simulink model "Crane_rigid"  (R2021b)
settings: Solver=ode15s  StartTime=0.0  StopTime=t_f  MaxStep=max_step_size  RelTol=1e-3
values from neighbouring files (symbols this model uses):
  a_d_full_y = circshift(a_d_full_x,floor(1/h))/2    [modify_tracking.m]
  cont_param_10 = in    [double_pendulum.m]    (also in optimize_10_SMC_single_first_explicit.m = cont_param_10_surrogateopt)
  cont_param_11 = in    [double_pendulum.m]    (also in optimize_11_SMC_single_first_implicit.m = cont_param_11_surrogateopt)
  cont_param_12 = in    [double_pendulum.m]    (also in optimize_12_SMC_single_last_explicit.m = cont_param_12_surrogateopt)
  cont_param_13 = in    [double_pendulum.m]    (also in optimize_13_SMC_single_last_implicit.m = cont_param_13_surrogateopt)
  cont_param_14 = in    [double_pendulum.m]    (also in optimize_14_SMC_double_explicit.m = cont_param_14_surrogateopt)
  cont_param_15 = in    [double_pendulum.m]    (also in optimize_15_SMC_double_implicit.m = cont_param_15_surrogateopt)
  cont_param_16 = in    [double_pendulum.m]
  cont_param_17 = in    [double_pendulum.m]
  cont_param_18 = in    [double_pendulum.m]
  cont_param_19 = in    [double_pendulum.m]
  cont_param_4 = in    [double_pendulum.m]
  cont_param_5 = in    [double_pendulum.m]
  cont_param_6 = in    [double_pendulum.m]
  cont_param_7 = in    [double_pendulum.m]
  cont_param_8 = in    [double_pendulum.m]
  cont_param_9 = in    [double_pendulum.m]
  h = 1e-5    (= 1e-05)    [Conference_paper.m]    (also in Latest.m)
  m = 10    [Conference_paper.m]    (also in Latest.m = 100; control_8_collocated_PD_tracking.m = load_mass+hook_mass+cable_mass_total)
  method_select = Method    [main_run.m]    (also in modify_tracking.m = 3)
  N = floor(t_f / h)    [control_2_zero_vibration.m]    (also in control_3_ZVD.m; modify_tracking.m = 3)
  s = c1*(x-xd)+c2*(v-vd)+c3*theta_dot_1+c4*theta_1    [control_10_SMC_single_first_explicit.m]    (also in control_11_SMC_single_first_implicit.m = c1*(x-xd)+c2*(v-vd)+c3*theta_dot+c4*theta; control_12_SMC_single_last_explicit.m = c1*(x-xd)+c2*(v-vd)+c3*theta_dot_2+c4*theta_2; control_13_SMC_single_last_implicit.m = c1*(x-xd)+c2*(v-vd)+c3*theta_dot+c4*theta; control_14_SMC_double_explicit.m = (v-vd)+lambda*(x-xd)+alpha*theta_1+beta*theta_2)
  sin_traj_w = 0.5    [modify_tracking.m]
  X = ex+lambda*sin(theta)    [control_16_PD_energy_first.m]    (also in control_17_PD_energy_last.m)
  Z = cont_param_8(4)    [control_8_collocated_PD_tracking.m]
undefined symbols (not defined in the file or in its folder): a_d_full_x, all_initial_sway, c_actuator, cable_length, cable_mass_total, cart_disturbance_amp, cart_mass, delay_time, first_link_sway, hook_mass, last_piece_length, load_disturbance_amp, number_of_pendulums, payload_mass, sat_const, sin_traj_A, t_f, total_mass, traj_number, unbalanced_factor, Y
libraries: nesl_utility x180, sm_lib x138, commchan3 x8
(part 2 of 3)

== system Crane_rigid/Rail ==
  F_x : Inport
  F_y : Inport  Port=2
  PS-Simulink Converter{,1..3} (4 alike) : nesl_utility/PS-Simulink Converter  PhysicalDomain=network_engine_domain  SubClassName=ps_output  LeftPortType=input  RightPortType=output  PseudoPeriodic=off  Frequencies=[]  Unit=inherit  AffineConversion=off
      settings: SourceProductBaseCode=PW,SS
  Rectangular Joint : sm_lib/Joints/Rectangular Joint  JointMode=Normal  SenseConstraintForce=off  SenseConstraintForceX=off  SenseConstraintForceY=off  SenseConstraintForceZ=off  SenseConstraintTorque=off  SenseConstraintTorqueX=off  SenseConstraintTorqueY=off  SenseConstraintTorqueZ=off  SenseTotalForce=off  SenseTotalForceX=off  SenseTotalForceY=off  SenseTotalForceZ=off  SenseTotalTorque=off  SenseTotalTorqueX=off  SenseTotalTorqueY=off  SenseTotalTorqueZ=off  CompositeWrenchDir=FollowerOnBase  CompositeWrenchFrame=BaseFrame  PxEquilibriumPosition=0  PxEquilibriumPositionUnits=m  PxSpringStiffness=0  PxSpringStiffnessUnits=N/m  PxDampingCoefficient=0  PxDampingCoefficientUnits=N/(m/s)  PxTorqueActuationMode=InputTorque  PxMotionActuationMode=ComputedMotion  PxSensePosition=off  PxSenseVelocity=off  PxSenseAcceleration=off  PxSenseTorqueForce=off  PxSenseLowerLimitTorqueForce=off  PxSenseUpperLimitTorqueForce=off  PxLowerLimitSpecify=off  PxLowerLimitBound=-1  PxLowerLimitBoundUnits=m  PxLowerLimitStiffness=1e6  PxLowerLimitStiffnessUnits=N/m  PxLowerLimitDamping=1e3  PxLowerLimitDampingUnits=N/(m/s)  PxLowerLimitTransitionRegionWidth=1e-4  PxLowerLimitTransitionRegionWidthUnits=m  PxUpperLimitSpecify=off  PxUpperLimitBound=1  PxUpperLimitBoundUnits=m  PxUpperLimitStiffness=1e6  PxUpperLimitStiffnessUnits=N/m  PxUpperLimitDamping=1e3  PxUpperLimitDampingUnits=N/(m/s)  PxUpperLimitTransitionRegionWidth=1e-4  PxUpperLimitTransitionRegionWidthUnits=m  PxPositionTargetSpecify=off  PxPositionTargetPriority=High  PxPositionTargetValue=0  PxPositionTargetValueUnits=m  PxVelocityTargetSpecify=off  PxVelocityTargetPriority=High  PxVelocityTargetValue=0  PxVelocityTargetValueUnits=m/s  PyEquilibriumPosition=0  PyEquilibriumPositionUnits=m  PySpringStiffness=0  PySpringStiffnessUnits=N/m  PyDampingCoefficient=0  PyDampingCoefficientUnits=N/(m/s)  PyTorqueActuationMode=InputTorque  PyMotionActuationMode=ComputedMotion  PySensePosition=off  PySenseVelocity=off  PySenseAcceleration=off  PySenseTorqueForce=off  PySenseLowerLimitTorqueForce=off  PySenseUpperLimitTorqueForce=off  PyLowerLimitSpecify=off  PyLowerLimitBound=-1  PyLowerLimitBoundUnits=m  PyLowerLimitStiffness=1e6  PyLowerLimitStiffnessUnits=N/m  PyLowerLimitDamping=1e3  PyLowerLimitDampingUnits=N/(m/s)  PyLowerLimitTransitionRegionWidth=1e-4  PyLowerLimitTransitionRegionWidthUnits=m  PyUpperLimitSpecify=off  PyUpperLimitBound=1  PyUpperLimitBoundUnits=m  PyUpperLimitStiffness=1e6  PyUpperLimitStiffnessUnits=N/m  PyUpperLimitDamping=1e3  PyUpperLimitDampingUnits=N/(m/s)  PyUpperLimitTransitionRegionWidth=1e-4  PyUpperLimitTransitionRegionWidthUnits=m  PyPositionTargetSpecify=off  PyPositionTargetPriority=High  PyPositionTargetValue=0  PyPositionTargetValueUnits=m  PyVelocityTargetSpecify=off  PyVelocityTargetPriority=High  PyVelocityTargetValue=0  PyVelocityTargetValueUnits=m/s
  Simulink-PS Converter1 : nesl_utility/Simulink-PS Converter  PhysicalDomain=network_engine_domain  SubClassName=ps_input  LeftPortType=input  RightPortType=output  PseudoPeriodic=off  Frequencies=[]  NoiseDistribution=none  NoiseParameters=[]  Unit=1  AffineConversion=off  FilteringAndDerivatives=provide  SimscapeFilterOrder=1  InputFilterTimeConstant=0.001  UdotUserProvided=0
      settings: SourceProductBaseCode=PW,SS
  Simulink-PS Converter2 : nesl_utility/Simulink-PS Converter  PhysicalDomain=network_engine_domain  SubClassName=ps_input  LeftPortType=input  RightPortType=output  PseudoPeriodic=off  Frequencies=[]  NoiseDistribution=none  NoiseParameters=[]  Unit=1  AffineConversion=off  FilteringAndDerivatives=provide  SimscapeFilterOrder=1  InputFilterTimeConstant=0.001  UdotUserProvided=0
      settings: SourceProductBaseCode=PW,SS
  Transform Sensor : sm_lib/Frames and Transforms/Transform Sensor  MeasurementFrame=World  SenseAngle=off  SenseAxis=off  SenseAngle1=off  SenseAngle2=off  SenseAngle3=off  SenseQ=off  SenseR=off  SenseOmegaX=off  SenseOmegaY=off  SenseOmegaZ=off  SenseOmega1=off  SenseOmega2=off  SenseOmega3=off  SenseQDot=off  SenseRDot=off  SenseAlphaX=off  SenseAlphaY=off  SenseAlphaZ=off  SenseAlpha1=off  SenseAlpha2=off  SenseAlpha3=off  SenseQDDot=off  SenseRDDot=off  SenseX=on  SenseY=on  SenseZ=off  SenseRad=off  SenseAzim=off  SenseDist=off  SenseInc=off  SenseXDot=on  SenseYDot=on  SenseZDot=off  SenseRadDot=off  SenseAzimDot=off  SenseDistDot=off  SenseIncDot=off  SenseXDDot=off  SenseYDDot=off  SenseZDDot=off  SenseRadDDot=off  SenseAzimDDot=off  SenseDistDDot=off  SenseIncDDot=off
  World Frame : sm_lib/Frames and Transforms/World Frame
  Connection Port : PMIOPort  Side=Left
  Connection Port1 : PMIOPort  Port=2  Side=Right
  tag scope: Trolley_position_x=global, Trolley_position_y=global, Trolley_velocity_x=global, Trolley_velocity_y=global
  wires:
  PS-Simulink Converter/1 -> [Trolley_position_x]  "Trolley_position_x"
  PS-Simulink Converter1/1 -> [Trolley_position_y]  "Trolley_position_y"
  PS-Simulink Converter2/1 -> [Trolley_velocity_x]  "Trolley_velocity_x"
  PS-Simulink Converter3/1 -> [Trolley_velocity_y]  "Trolley_velocity_y"
  F_x/1 -> Simulink-PS Converter1/1
  F_y/1 -> Simulink-PS Converter2/1
  connections:
  Connection Port/RConn1 -- Rectangular Joint/LConn1
  Connection Port1/RConn1 -- Rectangular Joint/RConn1 -- Transform Sensor/RConn1
  Transform Sensor/LConn1 -- World Frame/RConn1
  Transform Sensor/RConn2 -- PS-Simulink Converter/LConn1
  Transform Sensor/RConn3 -- PS-Simulink Converter1/LConn1
  Transform Sensor/RConn4 -- PS-Simulink Converter2/LConn1
  Transform Sensor/RConn5 -- PS-Simulink Converter3/LConn1
  Simulink-PS Converter1/RConn1 -- Rectangular Joint/LConn2
  Simulink-PS Converter2/RConn1 -- Rectangular Joint/LConn3

== system Crane_rigid/World Frame ==
  Mechanism Configuration : sm_lib/Utilities/Mechanism Configuration  UniformGravity=Constant  GravityVector=[0 0 -9.80665]  GravityUnits=m/s^2  LinearizationDelta=0.001  JointModeTransitionNonlinearIterations=2
  Solver Configuration : nesl_utility/Solver Configuration  PhysicalDomain=network_engine_domain  SubClassName=solver  LeftPortType=input  RightPortType=generic  Tones=[]  Harmonics=[]  SimulateNoise=off  Profile=off  UseLocalSampling=off  EnableSwitchedLinearOptims=on  FrequencyDomain=off  UseCCode=off  RelTol=0.001  AbsTol=1e-06  MinStep=1e-09  ToWorkspace=off  RevertToSquareIcSolve=off  NumHomotopyIterations=100  PhasorMode=off  PhasorModeNumHarmonics=1  DoDC=off  ResidualTolerance=1e-09  UseLocalSolver=off  LocalSolverChoice=NE_BACKWARD_EULER_ADVANCER  LocalSolverSampleTime=0.001  DoFixedCost=off  MaxNonlinIter=3  MaxModeIter=2  ComputeImpulses=off  ImpulseIterations=2  LinearAlgebra=auto  EquationFormulation=NE_TIME_EF  DelaysMemoryBudget=1024  AutomaticFiltering=on  FilteringTimeConstant=0.001  PartitionStorageMethod=AS_NEEDED  PartitionMemoryBudget=1024  PartitionMethod=ROBUST
      settings: SourceProductBaseCode=PW,SS
  World Frame : sm_lib/Frames and Transforms/World Frame
  Connection Port : PMIOPort  Side=Left
  connections:
  Solver Configuration/RConn1 -- Connection Port/RConn1 -- Mechanism Configuration/RConn1 -- World Frame/RConn1

== system Crane_rigid/trajectory generator ==
  Clock : Clock
  Clock1 : Clock
  Constant : Constant  Value=traj_number
  Constant1 : Constant  Value=traj_number
  Constant2 : Constant  Value=sin_traj_w
  Constant3 : Constant  Value=sin_traj_A
  Constant4 : Constant  Value=sin_traj_w
  Constant5 : Constant  Value=sin_traj_A
  Gain : Gain  Gain=0.5
  Gain1 : Gain  Gain=0.5
  Gain2 : Gain  Gain=0.5
  Transport Delay : TransportDelay
  Transport Delay1 : TransportDelay
  Transport Delay2 : TransportDelay
  traj1_y : MATLAB Function  TreatAsAtomicUnit=on
  traj_x : MATLAB Function  TreatAsAtomicUnit=on
  tag scope: xd=global, xd_ddot=global, xd_dot=global, yd=global, yd_ddot=global, yd_dot=global
  wires:
  traj_x/1(x_d) -> [xd]  "xd"
  Clock/1 -> traj_x/1(t)
  traj_x/2(v_d) -> [xd_dot]  "xd_dot"
  traj_x/3(a_d) -> [xd_ddot]  "xd_ddot"
  Constant/1 -> traj_x/2(traj_number)
  traj1_y/3(a_d) -> Gain2/1
  traj1_y/2(v_d) -> Gain1/1
  traj1_y/1(x_d) -> Gain/1
  Gain/1 -> Transport Delay/1
  Transport Delay/1 -> [yd]  "yd"
  Gain1/1 -> Transport Delay1/1
  Transport Delay1/1 -> [yd_dot]  "yd_dot"
  Gain2/1 -> Transport Delay2/1
  Transport Delay2/1 -> [yd_ddot]  "yd_ddot"
  Constant2/1 -> traj_x/3(sin_traj_w)
  Constant3/1 -> traj_x/4(sin_traj_A)
  Constant5/1 -> traj1_y/4(sin_traj_A)
  Constant4/1 -> traj1_y/3(sin_traj_w)
  Constant1/1 -> traj1_y/2(traj_number)
  Clock1/1 -> traj1_y/1(t)

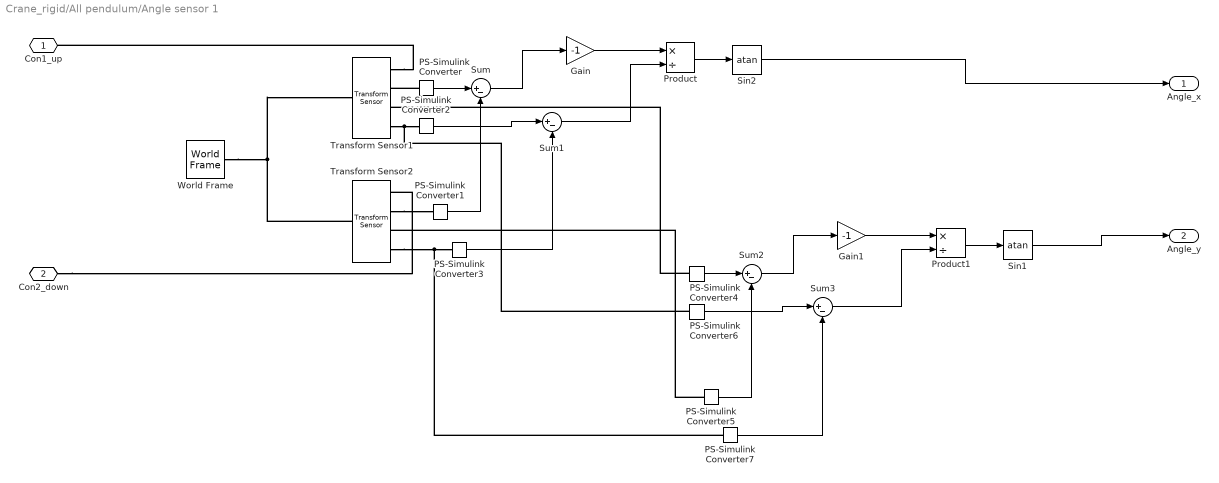
== system Crane_rigid/All pendulum/Angle sensor 1 ==
  Gain : Gain  Gain=-1
  Gain1 : Gain  Gain=-1
  PS-Simulink Converter{,1..7} (8 alike) : nesl_utility/PS-Simulink Converter  PhysicalDomain=network_engine_domain  SubClassName=ps_output  LeftPortType=input  RightPortType=output  PseudoPeriodic=off  Frequencies=[]  Unit=inherit  AffineConversion=off
      settings: SourceProductBaseCode=PW,SS
  Product : Product  Inputs=*/
  Product1 : Product  Inputs=*/
  Sin1 : Trigonometry  Operator=atan
  Sin2 : Trigonometry  Operator=atan
  Sum{,1..3} (4 alike) : Sum  Inputs=|+-
  Transform Sensor1 : sm_lib/Frames and Transforms/Transform Sensor  MeasurementFrame=World  SenseAngle=off  SenseAxis=off  SenseAngle1=off  SenseAngle2=off  SenseAngle3=off  SenseQ=off  SenseR=off  SenseOmegaX=off  SenseOmegaY=off  SenseOmegaZ=off  SenseOmega1=off  SenseOmega2=off  SenseOmega3=off  SenseQDot=off  SenseRDot=off  SenseAlphaX=off  SenseAlphaY=off  SenseAlphaZ=off  SenseAlpha1=off  SenseAlpha2=off  SenseAlpha3=off  SenseQDDot=off  SenseRDDot=off  SenseX=on  SenseY=on  SenseZ=on  SenseRad=off  SenseAzim=off  SenseDist=off  SenseInc=off  SenseXDot=off  SenseYDot=off  SenseZDot=off  SenseRadDot=off  SenseAzimDot=off  SenseDistDot=off  SenseIncDot=off  SenseXDDot=off  SenseYDDot=off  SenseZDDot=off  SenseRadDDot=off  SenseAzimDDot=off  SenseDistDDot=off  SenseIncDDot=off
  Transform Sensor2 : sm_lib/Frames and Transforms/Transform Sensor  MeasurementFrame=World  SenseAngle=off  SenseAxis=off  SenseAngle1=off  SenseAngle2=off  SenseAngle3=off  SenseQ=off  SenseR=off  SenseOmegaX=off  SenseOmegaY=off  SenseOmegaZ=off  SenseOmega1=off  SenseOmega2=off  SenseOmega3=off  SenseQDot=off  SenseRDot=off  SenseAlphaX=off  SenseAlphaY=off  SenseAlphaZ=off  SenseAlpha1=off  SenseAlpha2=off  SenseAlpha3=off  SenseQDDot=off  SenseRDDot=off  SenseX=on  SenseY=on  SenseZ=on  SenseRad=off  SenseAzim=off  SenseDist=off  SenseInc=off  SenseXDot=off  SenseYDot=off  SenseZDot=off  SenseRadDot=off  SenseAzimDot=off  SenseDistDot=off  SenseIncDot=off  SenseXDDot=off  SenseYDDot=off  SenseZDDot=off  SenseRadDDot=off  SenseAzimDDot=off  SenseDistDDot=off  SenseIncDDot=off
  World Frame : sm_lib/Frames and Transforms/World Frame
  Con1_up : PMIOPort  Side=Left
  Con2_down : PMIOPort  Port=2  Side=Left
  Angle_x : Outport
  Angle_y : Outport  Port=2
  wires:
  PS-Simulink Converter/1 -> Sum/1
  Sum1/1 -> Product/2
  Product/1 -> Sin2/1
  PS-Simulink Converter2/1 -> Sum1/1
  PS-Simulink Converter3/1 -> Sum1/2
  Gain/1 -> Product/1
  PS-Simulink Converter7/1 -> Sum3/2
  PS-Simulink Converter4/1 -> Sum2/1
  PS-Simulink Converter5/1 -> Sum2/2
  PS-Simulink Converter1/1 -> Sum/2
  PS-Simulink Converter6/1 -> Sum3/1
  Product1/1 -> Sin1/1
  Sum2/1 -> Gain1/1
  Sum3/1 -> Product1/2
  Gain1/1 -> Product1/1
  Sum/1 -> Gain/1
  Sin2/1 -> Angle_x/1
  Sin1/1 -> Angle_y/1
  connections:
  World Frame/RConn1 -- Transform Sensor2/LConn1 -- Transform Sensor1/LConn1
  Transform Sensor2/RConn4 -- PS-Simulink Converter7/LConn1 -- PS-Simulink Converter3/LConn1
  Transform Sensor1/RConn4 -- PS-Simulink Converter6/LConn1 -- PS-Simulink Converter2/LConn1
  PS-Simulink Converter5/LConn1 -- Transform Sensor2/RConn3
  PS-Simulink Converter4/LConn1 -- Transform Sensor1/RConn3
  Transform Sensor2/RConn2 -- PS-Simulink Converter1/LConn1
  PS-Simulink Converter/LConn1 -- Transform Sensor1/RConn2
  Transform Sensor1/RConn1 -- Con1_up/RConn1
  Con2_down/RConn1 -- Transform Sensor2/RConn1

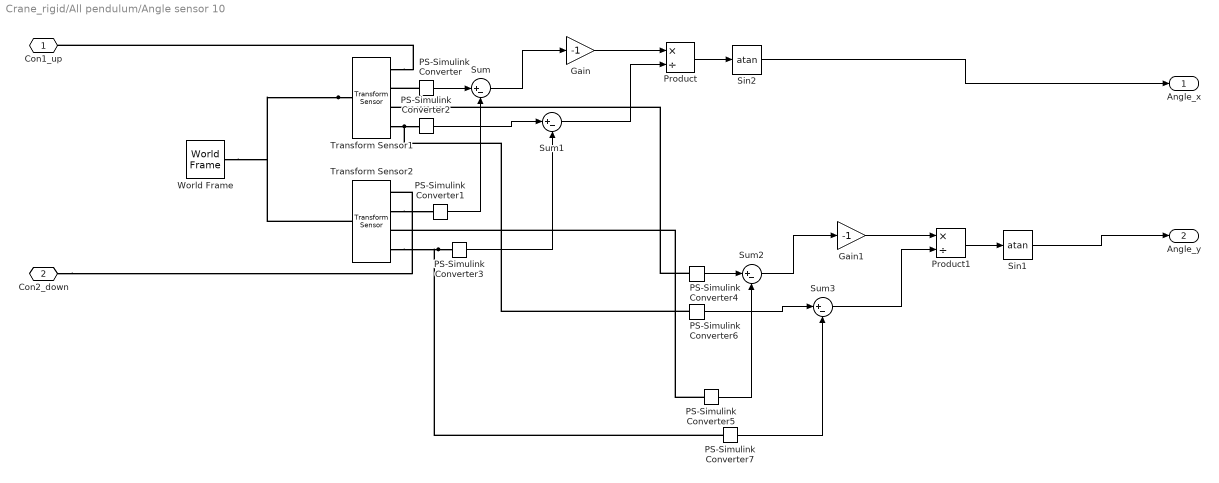
== system Crane_rigid/All pendulum/Angle sensor 10 ==
  Gain : Gain  Gain=-1
  Gain1 : Gain  Gain=-1
  PS-Simulink Converter{,1..7} (8 alike) : nesl_utility/PS-Simulink Converter  PhysicalDomain=network_engine_domain  SubClassName=ps_output  LeftPortType=input  RightPortType=output  PseudoPeriodic=off  Frequencies=[]  Unit=inherit  AffineConversion=off
      settings: SourceProductBaseCode=PW,SS
  Product : Product  Inputs=*/
  Product1 : Product  Inputs=*/
  Sin1 : Trigonometry  Operator=atan
  Sin2 : Trigonometry  Operator=atan
  Sum{,1..3} (4 alike) : Sum  Inputs=|+-
  Transform Sensor1 : sm_lib/Frames and Transforms/Transform Sensor  MeasurementFrame=World  SenseAngle=off  SenseAxis=off  SenseAngle1=off  SenseAngle2=off  SenseAngle3=off  SenseQ=off  SenseR=off  SenseOmegaX=off  SenseOmegaY=off  SenseOmegaZ=off  SenseOmega1=off  SenseOmega2=off  SenseOmega3=off  SenseQDot=off  SenseRDot=off  SenseAlphaX=off  SenseAlphaY=off  SenseAlphaZ=off  SenseAlpha1=off  SenseAlpha2=off  SenseAlpha3=off  SenseQDDot=off  SenseRDDot=off  SenseX=on  SenseY=on  SenseZ=on  SenseRad=off  SenseAzim=off  SenseDist=off  SenseInc=off  SenseXDot=off  SenseYDot=off  SenseZDot=off  SenseRadDot=off  SenseAzimDot=off  SenseDistDot=off  SenseIncDot=off  SenseXDDot=off  SenseYDDot=off  SenseZDDot=off  SenseRadDDot=off  SenseAzimDDot=off  SenseDistDDot=off  SenseIncDDot=off
  Transform Sensor2 : sm_lib/Frames and Transforms/Transform Sensor  MeasurementFrame=World  SenseAngle=off  SenseAxis=off  SenseAngle1=off  SenseAngle2=off  SenseAngle3=off  SenseQ=off  SenseR=off  SenseOmegaX=off  SenseOmegaY=off  SenseOmegaZ=off  SenseOmega1=off  SenseOmega2=off  SenseOmega3=off  SenseQDot=off  SenseRDot=off  SenseAlphaX=off  SenseAlphaY=off  SenseAlphaZ=off  SenseAlpha1=off  SenseAlpha2=off  SenseAlpha3=off  SenseQDDot=off  SenseRDDot=off  SenseX=on  SenseY=on  SenseZ=on  SenseRad=off  SenseAzim=off  SenseDist=off  SenseInc=off  SenseXDot=off  SenseYDot=off  SenseZDot=off  SenseRadDot=off  SenseAzimDot=off  SenseDistDot=off  SenseIncDot=off  SenseXDDot=off  SenseYDDot=off  SenseZDDot=off  SenseRadDDot=off  SenseAzimDDot=off  SenseDistDDot=off  SenseIncDDot=off
  World Frame : sm_lib/Frames and Transforms/World Frame
  Con1_up : PMIOPort  Side=Left
  Con2_down : PMIOPort  Port=2  Side=Left
  Angle_x : Outport
  Angle_y : Outport  Port=2
  wires:
  Sin1/1 -> Angle_y/1
  Sin2/1 -> Angle_x/1
  Sum/1 -> Gain/1
  Gain1/1 -> Product1/1
  Sum3/1 -> Product1/2
  Sum2/1 -> Gain1/1
  Product1/1 -> Sin1/1
  PS-Simulink Converter6/1 -> Sum3/1
  PS-Simulink Converter1/1 -> Sum/2
  PS-Simulink Converter5/1 -> Sum2/2
  PS-Simulink Converter4/1 -> Sum2/1
  PS-Simulink Converter7/1 -> Sum3/2
  Gain/1 -> Product/1
  PS-Simulink Converter3/1 -> Sum1/2
  PS-Simulink Converter2/1 -> Sum1/1
  Product/1 -> Sin2/1
  Sum1/1 -> Product/2
  PS-Simulink Converter/1 -> Sum/1
  connections:
  Con2_down/RConn1 -- Transform Sensor2/RConn1
  Transform Sensor1/RConn1 -- Con1_up/RConn1
  PS-Simulink Converter/LConn1 -- Transform Sensor1/RConn2
  Transform Sensor2/RConn2 -- PS-Simulink Converter1/LConn1
  PS-Simulink Converter4/LConn1 -- Transform Sensor1/RConn3
  PS-Simulink Converter5/LConn1 -- Transform Sensor2/RConn3
  PS-Simulink Converter2/LConn1 -- PS-Simulink Converter6/LConn1 -- Transform Sensor1/RConn4
  PS-Simulink Converter3/LConn1 -- PS-Simulink Converter7/LConn1 -- Transform Sensor2/RConn4
  Transform Sensor1/LConn1 -- Transform Sensor2/LConn1 -- World Frame/RConn1

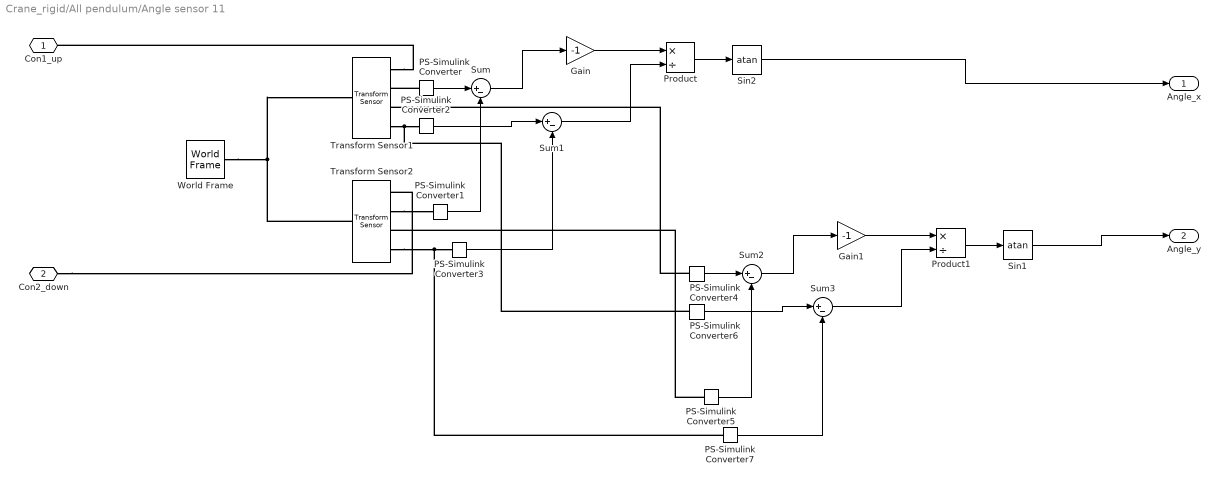
== system Crane_rigid/All pendulum/Angle sensor 11 ==
  Gain : Gain  Gain=-1
  Gain1 : Gain  Gain=-1
  PS-Simulink Converter{,1..7} (8 alike) : nesl_utility/PS-Simulink Converter  PhysicalDomain=network_engine_domain  SubClassName=ps_output  LeftPortType=input  RightPortType=output  PseudoPeriodic=off  Frequencies=[]  Unit=inherit  AffineConversion=off
      settings: SourceProductBaseCode=PW,SS
  Product : Product  Inputs=*/
  Product1 : Product  Inputs=*/
  Sin1 : Trigonometry  Operator=atan
  Sin2 : Trigonometry  Operator=atan
  Sum{,1..3} (4 alike) : Sum  Inputs=|+-
  Transform Sensor1 : sm_lib/Frames and Transforms/Transform Sensor  MeasurementFrame=World  SenseAngle=off  SenseAxis=off  SenseAngle1=off  SenseAngle2=off  SenseAngle3=off  SenseQ=off  SenseR=off  SenseOmegaX=off  SenseOmegaY=off  SenseOmegaZ=off  SenseOmega1=off  SenseOmega2=off  SenseOmega3=off  SenseQDot=off  SenseRDot=off  SenseAlphaX=off  SenseAlphaY=off  SenseAlphaZ=off  SenseAlpha1=off  SenseAlpha2=off  SenseAlpha3=off  SenseQDDot=off  SenseRDDot=off  SenseX=on  SenseY=on  SenseZ=on  SenseRad=off  SenseAzim=off  SenseDist=off  SenseInc=off  SenseXDot=off  SenseYDot=off  SenseZDot=off  SenseRadDot=off  SenseAzimDot=off  SenseDistDot=off  SenseIncDot=off  SenseXDDot=off  SenseYDDot=off  SenseZDDot=off  SenseRadDDot=off  SenseAzimDDot=off  SenseDistDDot=off  SenseIncDDot=off
  Transform Sensor2 : sm_lib/Frames and Transforms/Transform Sensor  MeasurementFrame=World  SenseAngle=off  SenseAxis=off  SenseAngle1=off  SenseAngle2=off  SenseAngle3=off  SenseQ=off  SenseR=off  SenseOmegaX=off  SenseOmegaY=off  SenseOmegaZ=off  SenseOmega1=off  SenseOmega2=off  SenseOmega3=off  SenseQDot=off  SenseRDot=off  SenseAlphaX=off  SenseAlphaY=off  SenseAlphaZ=off  SenseAlpha1=off  SenseAlpha2=off  SenseAlpha3=off  SenseQDDot=off  SenseRDDot=off  SenseX=on  SenseY=on  SenseZ=on  SenseRad=off  SenseAzim=off  SenseDist=off  SenseInc=off  SenseXDot=off  SenseYDot=off  SenseZDot=off  SenseRadDot=off  SenseAzimDot=off  SenseDistDot=off  SenseIncDot=off  SenseXDDot=off  SenseYDDot=off  SenseZDDot=off  SenseRadDDot=off  SenseAzimDDot=off  SenseDistDDot=off  SenseIncDDot=off
  World Frame : sm_lib/Frames and Transforms/World Frame
  Con1_up : PMIOPort  Side=Left
  Con2_down : PMIOPort  Port=2  Side=Left
  Angle_x : Outport
  Angle_y : Outport  Port=2
  wires:
  PS-Simulink Converter/1 -> Sum/1
  Sum1/1 -> Product/2
  Product/1 -> Sin2/1
  PS-Simulink Converter2/1 -> Sum1/1
  PS-Simulink Converter3/1 -> Sum1/2
  Gain/1 -> Product/1
  PS-Simulink Converter7/1 -> Sum3/2
  PS-Simulink Converter4/1 -> Sum2/1
  PS-Simulink Converter5/1 -> Sum2/2
  PS-Simulink Converter1/1 -> Sum/2
  PS-Simulink Converter6/1 -> Sum3/1
  Product1/1 -> Sin1/1
  Sum2/1 -> Gain1/1
  Sum3/1 -> Product1/2
  Gain1/1 -> Product1/1
  Sum/1 -> Gain/1
  Sin2/1 -> Angle_x/1
  Sin1/1 -> Angle_y/1
  connections:
  World Frame/RConn1 -- Transform Sensor2/LConn1 -- Transform Sensor1/LConn1
  Transform Sensor2/RConn4 -- PS-Simulink Converter7/LConn1 -- PS-Simulink Converter3/LConn1
  Transform Sensor1/RConn4 -- PS-Simulink Converter6/LConn1 -- PS-Simulink Converter2/LConn1
  PS-Simulink Converter5/LConn1 -- Transform Sensor2/RConn3
  PS-Simulink Converter4/LConn1 -- Transform Sensor1/RConn3
  Transform Sensor2/RConn2 -- PS-Simulink Converter1/LConn1
  PS-Simulink Converter/LConn1 -- Transform Sensor1/RConn2
  Transform Sensor1/RConn1 -- Con1_up/RConn1
  Con2_down/RConn1 -- Transform Sensor2/RConn1

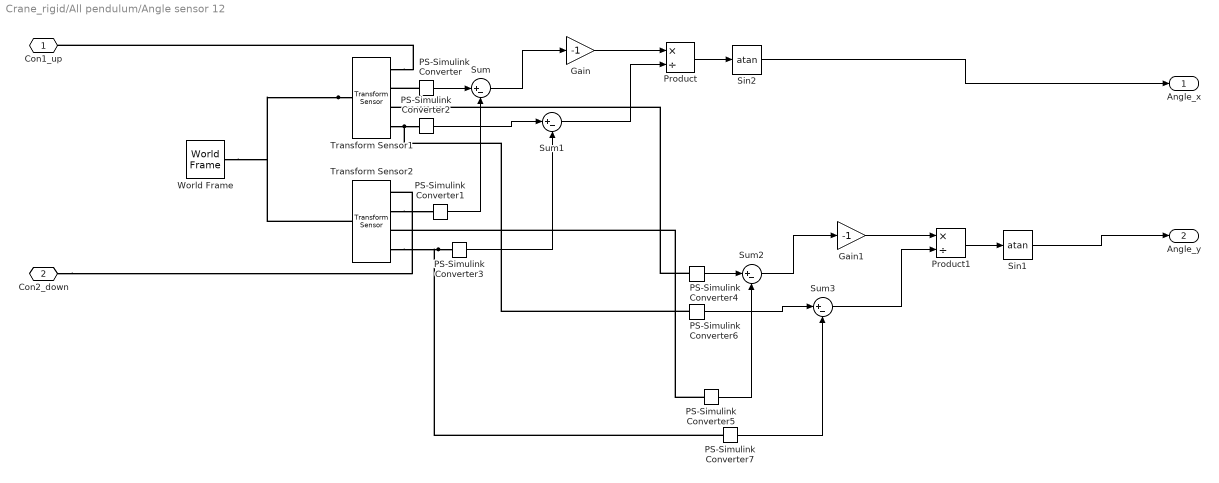
== system Crane_rigid/All pendulum/Angle sensor 12 ==
  Gain : Gain  Gain=-1
  Gain1 : Gain  Gain=-1
  PS-Simulink Converter{,1..7} (8 alike) : nesl_utility/PS-Simulink Converter  PhysicalDomain=network_engine_domain  SubClassName=ps_output  LeftPortType=input  RightPortType=output  PseudoPeriodic=off  Frequencies=[]  Unit=inherit  AffineConversion=off
      settings: SourceProductBaseCode=PW,SS
  Product : Product  Inputs=*/
  Product1 : Product  Inputs=*/
  Sin1 : Trigonometry  Operator=atan
  Sin2 : Trigonometry  Operator=atan
  Sum{,1..3} (4 alike) : Sum  Inputs=|+-
  Transform Sensor1 : sm_lib/Frames and Transforms/Transform Sensor  MeasurementFrame=World  SenseAngle=off  SenseAxis=off  SenseAngle1=off  SenseAngle2=off  SenseAngle3=off  SenseQ=off  SenseR=off  SenseOmegaX=off  SenseOmegaY=off  SenseOmegaZ=off  SenseOmega1=off  SenseOmega2=off  SenseOmega3=off  SenseQDot=off  SenseRDot=off  SenseAlphaX=off  SenseAlphaY=off  SenseAlphaZ=off  SenseAlpha1=off  SenseAlpha2=off  SenseAlpha3=off  SenseQDDot=off  SenseRDDot=off  SenseX=on  SenseY=on  SenseZ=on  SenseRad=off  SenseAzim=off  SenseDist=off  SenseInc=off  SenseXDot=off  SenseYDot=off  SenseZDot=off  SenseRadDot=off  SenseAzimDot=off  SenseDistDot=off  SenseIncDot=off  SenseXDDot=off  SenseYDDot=off  SenseZDDot=off  SenseRadDDot=off  SenseAzimDDot=off  SenseDistDDot=off  SenseIncDDot=off
  Transform Sensor2 : sm_lib/Frames and Transforms/Transform Sensor  MeasurementFrame=World  SenseAngle=off  SenseAxis=off  SenseAngle1=off  SenseAngle2=off  SenseAngle3=off  SenseQ=off  SenseR=off  SenseOmegaX=off  SenseOmegaY=off  SenseOmegaZ=off  SenseOmega1=off  SenseOmega2=off  SenseOmega3=off  SenseQDot=off  SenseRDot=off  SenseAlphaX=off  SenseAlphaY=off  SenseAlphaZ=off  SenseAlpha1=off  SenseAlpha2=off  SenseAlpha3=off  SenseQDDot=off  SenseRDDot=off  SenseX=on  SenseY=on  SenseZ=on  SenseRad=off  SenseAzim=off  SenseDist=off  SenseInc=off  SenseXDot=off  SenseYDot=off  SenseZDot=off  SenseRadDot=off  SenseAzimDot=off  SenseDistDot=off  SenseIncDot=off  SenseXDDot=off  SenseYDDot=off  SenseZDDot=off  SenseRadDDot=off  SenseAzimDDot=off  SenseDistDDot=off  SenseIncDDot=off
  World Frame : sm_lib/Frames and Transforms/World Frame
  Con1_up : PMIOPort  Side=Left
  Con2_down : PMIOPort  Port=2  Side=Left
  Angle_x : Outport
  Angle_y : Outport  Port=2
  wires:
  Sin1/1 -> Angle_y/1
  Sin2/1 -> Angle_x/1
  Sum/1 -> Gain/1
  Gain1/1 -> Product1/1
  Sum3/1 -> Product1/2
  Sum2/1 -> Gain1/1
  Product1/1 -> Sin1/1
  PS-Simulink Converter6/1 -> Sum3/1
  PS-Simulink Converter1/1 -> Sum/2
  PS-Simulink Converter5/1 -> Sum2/2
  PS-Simulink Converter4/1 -> Sum2/1
  PS-Simulink Converter7/1 -> Sum3/2
  Gain/1 -> Product/1
  PS-Simulink Converter3/1 -> Sum1/2
  PS-Simulink Converter2/1 -> Sum1/1
  Product/1 -> Sin2/1
  Sum1/1 -> Product/2
  PS-Simulink Converter/1 -> Sum/1
  connections:
  Con2_down/RConn1 -- Transform Sensor2/RConn1
  Transform Sensor1/RConn1 -- Con1_up/RConn1
  PS-Simulink Converter/LConn1 -- Transform Sensor1/RConn2
  Transform Sensor2/RConn2 -- PS-Simulink Converter1/LConn1
  PS-Simulink Converter4/LConn1 -- Transform Sensor1/RConn3
  PS-Simulink Converter5/LConn1 -- Transform Sensor2/RConn3
  PS-Simulink Converter2/LConn1 -- PS-Simulink Converter6/LConn1 -- Transform Sensor1/RConn4
  PS-Simulink Converter3/LConn1 -- PS-Simulink Converter7/LConn1 -- Transform Sensor2/RConn4
  Transform Sensor1/LConn1 -- Transform Sensor2/LConn1 -- World Frame/RConn1

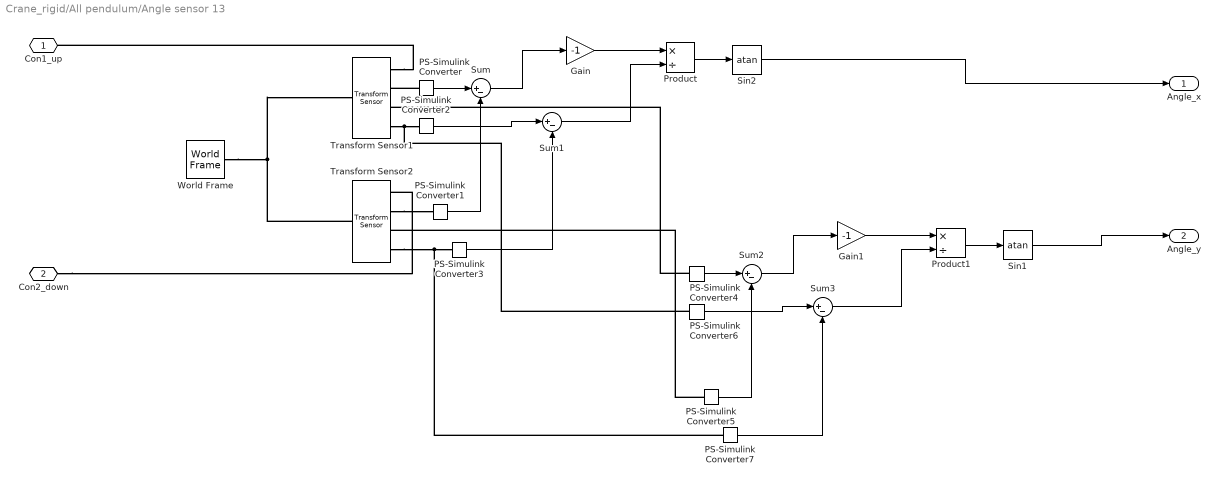
== system Crane_rigid/All pendulum/Angle sensor 13 ==
  Gain : Gain  Gain=-1
  Gain1 : Gain  Gain=-1
  PS-Simulink Converter{,1..7} (8 alike) : nesl_utility/PS-Simulink Converter  PhysicalDomain=network_engine_domain  SubClassName=ps_output  LeftPortType=input  RightPortType=output  PseudoPeriodic=off  Frequencies=[]  Unit=inherit  AffineConversion=off
      settings: SourceProductBaseCode=PW,SS
  Product : Product  Inputs=*/
  Product1 : Product  Inputs=*/
  Sin1 : Trigonometry  Operator=atan
  Sin2 : Trigonometry  Operator=atan
  Sum{,1..3} (4 alike) : Sum  Inputs=|+-
  Transform Sensor1 : sm_lib/Frames and Transforms/Transform Sensor  MeasurementFrame=World  SenseAngle=off  SenseAxis=off  SenseAngle1=off  SenseAngle2=off  SenseAngle3=off  SenseQ=off  SenseR=off  SenseOmegaX=off  SenseOmegaY=off  SenseOmegaZ=off  SenseOmega1=off  SenseOmega2=off  SenseOmega3=off  SenseQDot=off  SenseRDot=off  SenseAlphaX=off  SenseAlphaY=off  SenseAlphaZ=off  SenseAlpha1=off  SenseAlpha2=off  SenseAlpha3=off  SenseQDDot=off  SenseRDDot=off  SenseX=on  SenseY=on  SenseZ=on  SenseRad=off  SenseAzim=off  SenseDist=off  SenseInc=off  SenseXDot=off  SenseYDot=off  SenseZDot=off  SenseRadDot=off  SenseAzimDot=off  SenseDistDot=off  SenseIncDot=off  SenseXDDot=off  SenseYDDot=off  SenseZDDot=off  SenseRadDDot=off  SenseAzimDDot=off  SenseDistDDot=off  SenseIncDDot=off
  Transform Sensor2 : sm_lib/Frames and Transforms/Transform Sensor  MeasurementFrame=World  SenseAngle=off  SenseAxis=off  SenseAngle1=off  SenseAngle2=off  SenseAngle3=off  SenseQ=off  SenseR=off  SenseOmegaX=off  SenseOmegaY=off  SenseOmegaZ=off  SenseOmega1=off  SenseOmega2=off  SenseOmega3=off  SenseQDot=off  SenseRDot=off  SenseAlphaX=off  SenseAlphaY=off  SenseAlphaZ=off  SenseAlpha1=off  SenseAlpha2=off  SenseAlpha3=off  SenseQDDot=off  SenseRDDot=off  SenseX=on  SenseY=on  SenseZ=on  SenseRad=off  SenseAzim=off  SenseDist=off  SenseInc=off  SenseXDot=off  SenseYDot=off  SenseZDot=off  SenseRadDot=off  SenseAzimDot=off  SenseDistDot=off  SenseIncDot=off  SenseXDDot=off  SenseYDDot=off  SenseZDDot=off  SenseRadDDot=off  SenseAzimDDot=off  SenseDistDDot=off  SenseIncDDot=off
  World Frame : sm_lib/Frames and Transforms/World Frame
  Con1_up : PMIOPort  Side=Left
  Con2_down : PMIOPort  Port=2  Side=Left
  Angle_x : Outport
  Angle_y : Outport  Port=2
  wires:
  PS-Simulink Converter/1 -> Sum/1
  Sum1/1 -> Product/2
  Product/1 -> Sin2/1
  PS-Simulink Converter2/1 -> Sum1/1
  PS-Simulink Converter3/1 -> Sum1/2
  Gain/1 -> Product/1
  PS-Simulink Converter7/1 -> Sum3/2
  PS-Simulink Converter4/1 -> Sum2/1
  PS-Simulink Converter5/1 -> Sum2/2
  PS-Simulink Converter1/1 -> Sum/2
  PS-Simulink Converter6/1 -> Sum3/1
  Product1/1 -> Sin1/1
  Sum2/1 -> Gain1/1
  Sum3/1 -> Product1/2
  Gain1/1 -> Product1/1
  Sum/1 -> Gain/1
  Sin2/1 -> Angle_x/1
  Sin1/1 -> Angle_y/1
  connections:
  World Frame/RConn1 -- Transform Sensor2/LConn1 -- Transform Sensor1/LConn1
  Transform Sensor2/RConn4 -- PS-Simulink Converter7/LConn1 -- PS-Simulink Converter3/LConn1
  Transform Sensor1/RConn4 -- PS-Simulink Converter6/LConn1 -- PS-Simulink Converter2/LConn1
  PS-Simulink Converter5/LConn1 -- Transform Sensor2/RConn3
  PS-Simulink Converter4/LConn1 -- Transform Sensor1/RConn3
  Transform Sensor2/RConn2 -- PS-Simulink Converter1/LConn1
  PS-Simulink Converter/LConn1 -- Transform Sensor1/RConn2
  Transform Sensor1/RConn1 -- Con1_up/RConn1
  Con2_down/RConn1 -- Transform Sensor2/RConn1

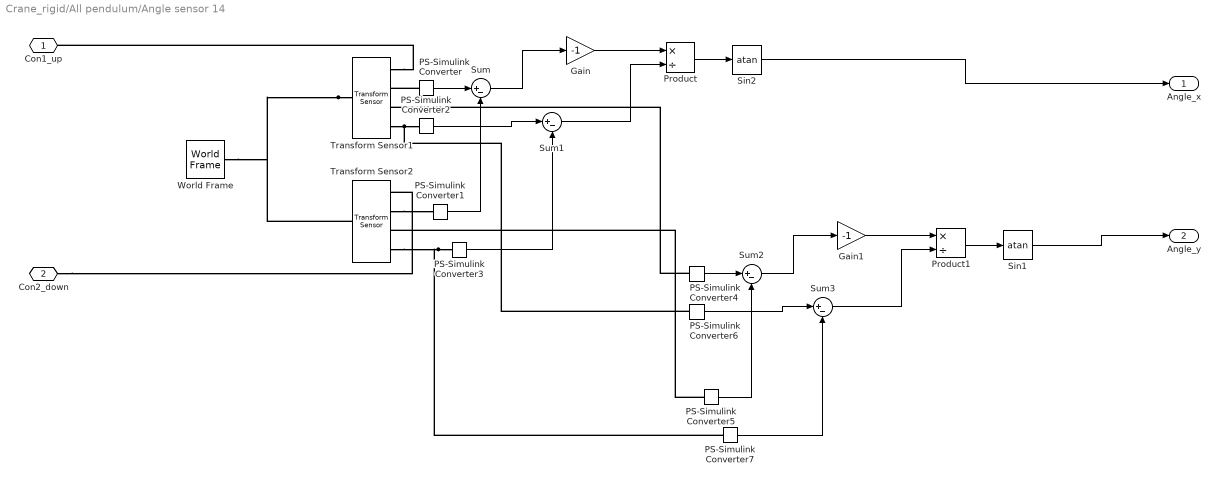
== system Crane_rigid/All pendulum/Angle sensor 14 ==
  Gain : Gain  Gain=-1
  Gain1 : Gain  Gain=-1
  PS-Simulink Converter{,1..7} (8 alike) : nesl_utility/PS-Simulink Converter  PhysicalDomain=network_engine_domain  SubClassName=ps_output  LeftPortType=input  RightPortType=output  PseudoPeriodic=off  Frequencies=[]  Unit=inherit  AffineConversion=off
      settings: SourceProductBaseCode=PW,SS
  Product : Product  Inputs=*/
  Product1 : Product  Inputs=*/
  Sin1 : Trigonometry  Operator=atan
  Sin2 : Trigonometry  Operator=atan
  Sum{,1..3} (4 alike) : Sum  Inputs=|+-
  Transform Sensor1 : sm_lib/Frames and Transforms/Transform Sensor  MeasurementFrame=World  SenseAngle=off  SenseAxis=off  SenseAngle1=off  SenseAngle2=off  SenseAngle3=off  SenseQ=off  SenseR=off  SenseOmegaX=off  SenseOmegaY=off  SenseOmegaZ=off  SenseOmega1=off  SenseOmega2=off  SenseOmega3=off  SenseQDot=off  SenseRDot=off  SenseAlphaX=off  SenseAlphaY=off  SenseAlphaZ=off  SenseAlpha1=off  SenseAlpha2=off  SenseAlpha3=off  SenseQDDot=off  SenseRDDot=off  SenseX=on  SenseY=on  SenseZ=on  SenseRad=off  SenseAzim=off  SenseDist=off  SenseInc=off  SenseXDot=off  SenseYDot=off  SenseZDot=off  SenseRadDot=off  SenseAzimDot=off  SenseDistDot=off  SenseIncDot=off  SenseXDDot=off  SenseYDDot=off  SenseZDDot=off  SenseRadDDot=off  SenseAzimDDot=off  SenseDistDDot=off  SenseIncDDot=off
  Transform Sensor2 : sm_lib/Frames and Transforms/Transform Sensor  MeasurementFrame=World  SenseAngle=off  SenseAxis=off  SenseAngle1=off  SenseAngle2=off  SenseAngle3=off  SenseQ=off  SenseR=off  SenseOmegaX=off  SenseOmegaY=off  SenseOmegaZ=off  SenseOmega1=off  SenseOmega2=off  SenseOmega3=off  SenseQDot=off  SenseRDot=off  SenseAlphaX=off  SenseAlphaY=off  SenseAlphaZ=off  SenseAlpha1=off  SenseAlpha2=off  SenseAlpha3=off  SenseQDDot=off  SenseRDDot=off  SenseX=on  SenseY=on  SenseZ=on  SenseRad=off  SenseAzim=off  SenseDist=off  SenseInc=off  SenseXDot=off  SenseYDot=off  SenseZDot=off  SenseRadDot=off  SenseAzimDot=off  SenseDistDot=off  SenseIncDot=off  SenseXDDot=off  SenseYDDot=off  SenseZDDot=off  SenseRadDDot=off  SenseAzimDDot=off  SenseDistDDot=off  SenseIncDDot=off
  World Frame : sm_lib/Frames and Transforms/World Frame
  Con1_up : PMIOPort  Side=Left
  Con2_down : PMIOPort  Port=2  Side=Left
  Angle_x : Outport
  Angle_y : Outport  Port=2
  wires:
  Sin1/1 -> Angle_y/1
  Sin2/1 -> Angle_x/1
  Sum/1 -> Gain/1
  Gain1/1 -> Product1/1
  Sum3/1 -> Product1/2
  Sum2/1 -> Gain1/1
  Product1/1 -> Sin1/1
  PS-Simulink Converter6/1 -> Sum3/1
  PS-Simulink Converter1/1 -> Sum/2
  PS-Simulink Converter5/1 -> Sum2/2
  PS-Simulink Converter4/1 -> Sum2/1
  PS-Simulink Converter7/1 -> Sum3/2
  Gain/1 -> Product/1
  PS-Simulink Converter3/1 -> Sum1/2
  PS-Simulink Converter2/1 -> Sum1/1
  Product/1 -> Sin2/1
  Sum1/1 -> Product/2
  PS-Simulink Converter/1 -> Sum/1
  connections:
  Con2_down/RConn1 -- Transform Sensor2/RConn1
  Transform Sensor1/RConn1 -- Con1_up/RConn1
  PS-Simulink Converter/LConn1 -- Transform Sensor1/RConn2
  Transform Sensor2/RConn2 -- PS-Simulink Converter1/LConn1
  PS-Simulink Converter4/LConn1 -- Transform Sensor1/RConn3
  PS-Simulink Converter5/LConn1 -- Transform Sensor2/RConn3
  PS-Simulink Converter2/LConn1 -- PS-Simulink Converter6/LConn1 -- Transform Sensor1/RConn4
  PS-Simulink Converter3/LConn1 -- PS-Simulink Converter7/LConn1 -- Transform Sensor2/RConn4
  Transform Sensor1/LConn1 -- Transform Sensor2/LConn1 -- World Frame/RConn1

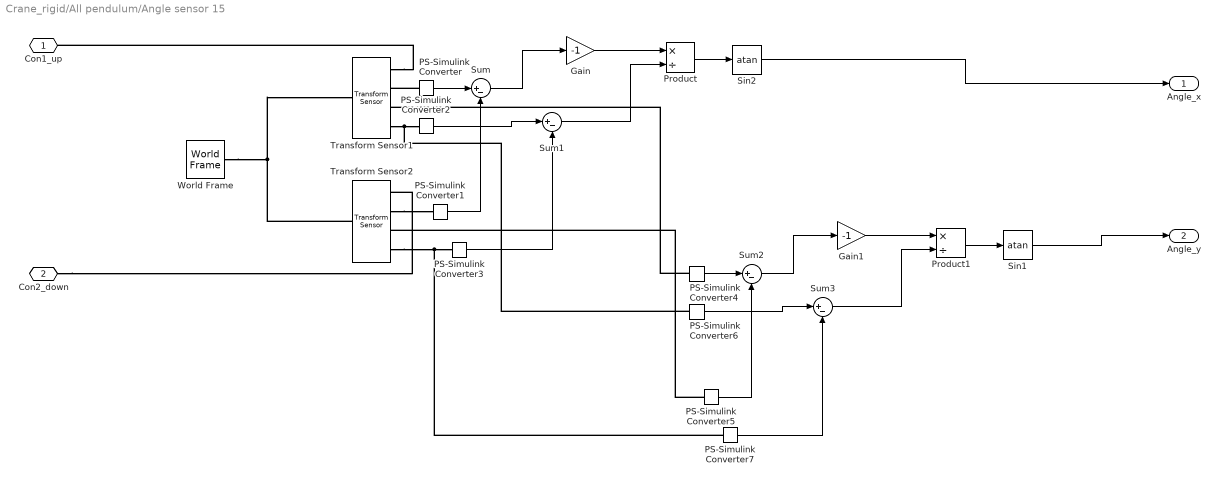
== system Crane_rigid/All pendulum/Angle sensor 15 ==
  Gain : Gain  Gain=-1
  Gain1 : Gain  Gain=-1
  PS-Simulink Converter{,1..7} (8 alike) : nesl_utility/PS-Simulink Converter  PhysicalDomain=network_engine_domain  SubClassName=ps_output  LeftPortType=input  RightPortType=output  PseudoPeriodic=off  Frequencies=[]  Unit=inherit  AffineConversion=off
      settings: SourceProductBaseCode=PW,SS
  Product : Product  Inputs=*/
  Product1 : Product  Inputs=*/
  Sin1 : Trigonometry  Operator=atan
  Sin2 : Trigonometry  Operator=atan
  Sum{,1..3} (4 alike) : Sum  Inputs=|+-
  Transform Sensor1 : sm_lib/Frames and Transforms/Transform Sensor  MeasurementFrame=World  SenseAngle=off  SenseAxis=off  SenseAngle1=off  SenseAngle2=off  SenseAngle3=off  SenseQ=off  SenseR=off  SenseOmegaX=off  SenseOmegaY=off  SenseOmegaZ=off  SenseOmega1=off  SenseOmega2=off  SenseOmega3=off  SenseQDot=off  SenseRDot=off  SenseAlphaX=off  SenseAlphaY=off  SenseAlphaZ=off  SenseAlpha1=off  SenseAlpha2=off  SenseAlpha3=off  SenseQDDot=off  SenseRDDot=off  SenseX=on  SenseY=on  SenseZ=on  SenseRad=off  SenseAzim=off  SenseDist=off  SenseInc=off  SenseXDot=off  SenseYDot=off  SenseZDot=off  SenseRadDot=off  SenseAzimDot=off  SenseDistDot=off  SenseIncDot=off  SenseXDDot=off  SenseYDDot=off  SenseZDDot=off  SenseRadDDot=off  SenseAzimDDot=off  SenseDistDDot=off  SenseIncDDot=off
  Transform Sensor2 : sm_lib/Frames and Transforms/Transform Sensor  MeasurementFrame=World  SenseAngle=off  SenseAxis=off  SenseAngle1=off  SenseAngle2=off  SenseAngle3=off  SenseQ=off  SenseR=off  SenseOmegaX=off  SenseOmegaY=off  SenseOmegaZ=off  SenseOmega1=off  SenseOmega2=off  SenseOmega3=off  SenseQDot=off  SenseRDot=off  SenseAlphaX=off  SenseAlphaY=off  SenseAlphaZ=off  SenseAlpha1=off  SenseAlpha2=off  SenseAlpha3=off  SenseQDDot=off  SenseRDDot=off  SenseX=on  SenseY=on  SenseZ=on  SenseRad=off  SenseAzim=off  SenseDist=off  SenseInc=off  SenseXDot=off  SenseYDot=off  SenseZDot=off  SenseRadDot=off  SenseAzimDot=off  SenseDistDot=off  SenseIncDot=off  SenseXDDot=off  SenseYDDot=off  SenseZDDot=off  SenseRadDDot=off  SenseAzimDDot=off  SenseDistDDot=off  SenseIncDDot=off
  World Frame : sm_lib/Frames and Transforms/World Frame
  Con1_up : PMIOPort  Side=Left
  Con2_down : PMIOPort  Port=2  Side=Left
  Angle_x : Outport
  Angle_y : Outport  Port=2
  wires:
  PS-Simulink Converter/1 -> Sum/1
  Sum1/1 -> Product/2
  Product/1 -> Sin2/1
  PS-Simulink Converter2/1 -> Sum1/1
  PS-Simulink Converter3/1 -> Sum1/2
  Gain/1 -> Product/1
  PS-Simulink Converter7/1 -> Sum3/2
  PS-Simulink Converter4/1 -> Sum2/1
  PS-Simulink Converter5/1 -> Sum2/2
  PS-Simulink Converter1/1 -> Sum/2
  PS-Simulink Converter6/1 -> Sum3/1
  Product1/1 -> Sin1/1
  Sum2/1 -> Gain1/1
  Sum3/1 -> Product1/2
  Gain1/1 -> Product1/1
  Sum/1 -> Gain/1
  Sin2/1 -> Angle_x/1
  Sin1/1 -> Angle_y/1
  connections:
  World Frame/RConn1 -- Transform Sensor2/LConn1 -- Transform Sensor1/LConn1
  Transform Sensor2/RConn4 -- PS-Simulink Converter7/LConn1 -- PS-Simulink Converter3/LConn1
  Transform Sensor1/RConn4 -- PS-Simulink Converter6/LConn1 -- PS-Simulink Converter2/LConn1
  PS-Simulink Converter5/LConn1 -- Transform Sensor2/RConn3
  PS-Simulink Converter4/LConn1 -- Transform Sensor1/RConn3
  Transform Sensor2/RConn2 -- PS-Simulink Converter1/LConn1
  PS-Simulink Converter/LConn1 -- Transform Sensor1/RConn2
  Transform Sensor1/RConn1 -- Con1_up/RConn1
  Con2_down/RConn1 -- Transform Sensor2/RConn1

== system Crane_rigid/All pendulum/Angle sensor 16 ==
  Gain : Gain  Gain=-1
  Gain1 : Gain  Gain=-1
  PS-Simulink Converter{,1..7} (8 alike) : nesl_utility/PS-Simulink Converter  PhysicalDomain=network_engine_domain  SubClassName=ps_output  LeftPortType=input  RightPortType=output  PseudoPeriodic=off  Frequencies=[]  Unit=inherit  AffineConversion=off
      settings: SourceProductBaseCode=PW,SS
  Product : Product  Inputs=*/
  Product1 : Product  Inputs=*/
  Sin1 : Trigonometry  Operator=atan
  Sin2 : Trigonometry  Operator=atan
  Sum{,1..3} (4 alike) : Sum  Inputs=|+-
  Transform Sensor1 : sm_lib/Frames and Transforms/Transform Sensor  MeasurementFrame=World  SenseAngle=off  SenseAxis=off  SenseAngle1=off  SenseAngle2=off  SenseAngle3=off  SenseQ=off  SenseR=off  SenseOmegaX=off  SenseOmegaY=off  SenseOmegaZ=off  SenseOmega1=off  SenseOmega2=off  SenseOmega3=off  SenseQDot=off  SenseRDot=off  SenseAlphaX=off  SenseAlphaY=off  SenseAlphaZ=off  SenseAlpha1=off  SenseAlpha2=off  SenseAlpha3=off  SenseQDDot=off  SenseRDDot=off  SenseX=on  SenseY=on  SenseZ=on  SenseRad=off  SenseAzim=off  SenseDist=off  SenseInc=off  SenseXDot=off  SenseYDot=off  SenseZDot=off  SenseRadDot=off  SenseAzimDot=off  SenseDistDot=off  SenseIncDot=off  SenseXDDot=off  SenseYDDot=off  SenseZDDot=off  SenseRadDDot=off  SenseAzimDDot=off  SenseDistDDot=off  SenseIncDDot=off
  Transform Sensor2 : sm_lib/Frames and Transforms/Transform Sensor  MeasurementFrame=World  SenseAngle=off  SenseAxis=off  SenseAngle1=off  SenseAngle2=off  SenseAngle3=off  SenseQ=off  SenseR=off  SenseOmegaX=off  SenseOmegaY=off  SenseOmegaZ=off  SenseOmega1=off  SenseOmega2=off  SenseOmega3=off  SenseQDot=off  SenseRDot=off  SenseAlphaX=off  SenseAlphaY=off  SenseAlphaZ=off  SenseAlpha1=off  SenseAlpha2=off  SenseAlpha3=off  SenseQDDot=off  SenseRDDot=off  SenseX=on  SenseY=on  SenseZ=on  SenseRad=off  SenseAzim=off  SenseDist=off  SenseInc=off  SenseXDot=off  SenseYDot=off  SenseZDot=off  SenseRadDot=off  SenseAzimDot=off  SenseDistDot=off  SenseIncDot=off  SenseXDDot=off  SenseYDDot=off  SenseZDDot=off  SenseRadDDot=off  SenseAzimDDot=off  SenseDistDDot=off  SenseIncDDot=off
  World Frame : sm_lib/Frames and Transforms/World Frame
  Con1_up : PMIOPort  Side=Left
  Con2_down : PMIOPort  Port=2  Side=Left
  Angle_x : Outport
  Angle_y : Outport  Port=2
  wires:
  Sin1/1 -> Angle_y/1
  Sin2/1 -> Angle_x/1
  Sum/1 -> Gain/1
  Gain1/1 -> Product1/1
  Sum3/1 -> Product1/2
  Sum2/1 -> Gain1/1
  Product1/1 -> Sin1/1
  PS-Simulink Converter6/1 -> Sum3/1
  PS-Simulink Converter1/1 -> Sum/2
  PS-Simulink Converter5/1 -> Sum2/2
  PS-Simulink Converter4/1 -> Sum2/1
  PS-Simulink Converter7/1 -> Sum3/2
  Gain/1 -> Product/1
  PS-Simulink Converter3/1 -> Sum1/2
  PS-Simulink Converter2/1 -> Sum1/1
  Product/1 -> Sin2/1
  Sum1/1 -> Product/2
  PS-Simulink Converter/1 -> Sum/1
  connections:
  Con2_down/RConn1 -- Transform Sensor2/RConn1
  Transform Sensor1/RConn1 -- Con1_up/RConn1
  PS-Simulink Converter/LConn1 -- Transform Sensor1/RConn2
  Transform Sensor2/RConn2 -- PS-Simulink Converter1/LConn1
  PS-Simulink Converter4/LConn1 -- Transform Sensor1/RConn3
  PS-Simulink Converter5/LConn1 -- Transform Sensor2/RConn3
  PS-Simulink Converter2/LConn1 -- PS-Simulink Converter6/LConn1 -- Transform Sensor1/RConn4
  PS-Simulink Converter3/LConn1 -- PS-Simulink Converter7/LConn1 -- Transform Sensor2/RConn4
  Transform Sensor1/LConn1 -- Transform Sensor2/LConn1 -- World Frame/RConn1

== system Crane_rigid/All pendulum/Angle sensor 17 ==
  Gain : Gain  Gain=-1
  Gain1 : Gain  Gain=-1
  PS-Simulink Converter{,1..7} (8 alike) : nesl_utility/PS-Simulink Converter  PhysicalDomain=network_engine_domain  SubClassName=ps_output  LeftPortType=input  RightPortType=output  PseudoPeriodic=off  Frequencies=[]  Unit=inherit  AffineConversion=off
      settings: SourceProductBaseCode=PW,SS
  Product : Product  Inputs=*/
  Product1 : Product  Inputs=*/
  Sin1 : Trigonometry  Operator=atan
  Sin2 : Trigonometry  Operator=atan
  Sum{,1..3} (4 alike) : Sum  Inputs=|+-
  Transform Sensor1 : sm_lib/Frames and Transforms/Transform Sensor  MeasurementFrame=World  SenseAngle=off  SenseAxis=off  SenseAngle1=off  SenseAngle2=off  SenseAngle3=off  SenseQ=off  SenseR=off  SenseOmegaX=off  SenseOmegaY=off  SenseOmegaZ=off  SenseOmega1=off  SenseOmega2=off  SenseOmega3=off  SenseQDot=off  SenseRDot=off  SenseAlphaX=off  SenseAlphaY=off  SenseAlphaZ=off  SenseAlpha1=off  SenseAlpha2=off  SenseAlpha3=off  SenseQDDot=off  SenseRDDot=off  SenseX=on  SenseY=on  SenseZ=on  SenseRad=off  SenseAzim=off  SenseDist=off  SenseInc=off  SenseXDot=off  SenseYDot=off  SenseZDot=off  SenseRadDot=off  SenseAzimDot=off  SenseDistDot=off  SenseIncDot=off  SenseXDDot=off  SenseYDDot=off  SenseZDDot=off  SenseRadDDot=off  SenseAzimDDot=off  SenseDistDDot=off  SenseIncDDot=off
  Transform Sensor2 : sm_lib/Frames and Transforms/Transform Sensor  MeasurementFrame=World  SenseAngle=off  SenseAxis=off  SenseAngle1=off  SenseAngle2=off  SenseAngle3=off  SenseQ=off  SenseR=off  SenseOmegaX=off  SenseOmegaY=off  SenseOmegaZ=off  SenseOmega1=off  SenseOmega2=off  SenseOmega3=off  SenseQDot=off  SenseRDot=off  SenseAlphaX=off  SenseAlphaY=off  SenseAlphaZ=off  SenseAlpha1=off  SenseAlpha2=off  SenseAlpha3=off  SenseQDDot=off  SenseRDDot=off  SenseX=on  SenseY=on  SenseZ=on  SenseRad=off  SenseAzim=off  SenseDist=off  SenseInc=off  SenseXDot=off  SenseYDot=off  SenseZDot=off  SenseRadDot=off  SenseAzimDot=off  SenseDistDot=off  SenseIncDot=off  SenseXDDot=off  SenseYDDot=off  SenseZDDot=off  SenseRadDDot=off  SenseAzimDDot=off  SenseDistDDot=off  SenseIncDDot=off
  World Frame : sm_lib/Frames and Transforms/World Frame
  Con1_up : PMIOPort  Side=Left
  Con2_down : PMIOPort  Port=2  Side=Left
  Angle_x : Outport
  Angle_y : Outport  Port=2
  wires:
  PS-Simulink Converter/1 -> Sum/1
  Sum1/1 -> Product/2
  Product/1 -> Sin2/1
  PS-Simulink Converter2/1 -> Sum1/1
  PS-Simulink Converter3/1 -> Sum1/2
  Gain/1 -> Product/1
  PS-Simulink Converter7/1 -> Sum3/2
  PS-Simulink Converter4/1 -> Sum2/1
  PS-Simulink Converter5/1 -> Sum2/2
  PS-Simulink Converter1/1 -> Sum/2
  PS-Simulink Converter6/1 -> Sum3/1
  Product1/1 -> Sin1/1
  Sum2/1 -> Gain1/1
  Sum3/1 -> Product1/2
  Gain1/1 -> Product1/1
  Sum/1 -> Gain/1
  Sin2/1 -> Angle_x/1
  Sin1/1 -> Angle_y/1
  connections:
  World Frame/RConn1 -- Transform Sensor2/LConn1 -- Transform Sensor1/LConn1
  Transform Sensor2/RConn4 -- PS-Simulink Converter7/LConn1 -- PS-Simulink Converter3/LConn1
  Transform Sensor1/RConn4 -- PS-Simulink Converter6/LConn1 -- PS-Simulink Converter2/LConn1
  PS-Simulink Converter5/LConn1 -- Transform Sensor2/RConn3
  PS-Simulink Converter4/LConn1 -- Transform Sensor1/RConn3
  Transform Sensor2/RConn2 -- PS-Simulink Converter1/LConn1
  PS-Simulink Converter/LConn1 -- Transform Sensor1/RConn2
  Transform Sensor1/RConn1 -- Con1_up/RConn1
  Con2_down/RConn1 -- Transform Sensor2/RConn1

== system Crane_rigid/All pendulum/Angle sensor 18 ==
  Gain : Gain  Gain=-1
  Gain1 : Gain  Gain=-1
  PS-Simulink Converter{,1..7} (8 alike) : nesl_utility/PS-Simulink Converter  PhysicalDomain=network_engine_domain  SubClassName=ps_output  LeftPortType=input  RightPortType=output  PseudoPeriodic=off  Frequencies=[]  Unit=inherit  AffineConversion=off
      settings: SourceProductBaseCode=PW,SS
  Product : Product  Inputs=*/
  Product1 : Product  Inputs=*/
  Sin1 : Trigonometry  Operator=atan
  Sin2 : Trigonometry  Operator=atan
  Sum{,1..3} (4 alike) : Sum  Inputs=|+-
  Transform Sensor1 : sm_lib/Frames and Transforms/Transform Sensor  MeasurementFrame=World  SenseAngle=off  SenseAxis=off  SenseAngle1=off  SenseAngle2=off  SenseAngle3=off  SenseQ=off  SenseR=off  SenseOmegaX=off  SenseOmegaY=off  SenseOmegaZ=off  SenseOmega1=off  SenseOmega2=off  SenseOmega3=off  SenseQDot=off  SenseRDot=off  SenseAlphaX=off  SenseAlphaY=off  SenseAlphaZ=off  SenseAlpha1=off  SenseAlpha2=off  SenseAlpha3=off  SenseQDDot=off  SenseRDDot=off  SenseX=on  SenseY=on  SenseZ=on  SenseRad=off  SenseAzim=off  SenseDist=off  SenseInc=off  SenseXDot=off  SenseYDot=off  SenseZDot=off  SenseRadDot=off  SenseAzimDot=off  SenseDistDot=off  SenseIncDot=off  SenseXDDot=off  SenseYDDot=off  SenseZDDot=off  SenseRadDDot=off  SenseAzimDDot=off  SenseDistDDot=off  SenseIncDDot=off
  Transform Sensor2 : sm_lib/Frames and Transforms/Transform Sensor  MeasurementFrame=World  SenseAngle=off  SenseAxis=off  SenseAngle1=off  SenseAngle2=off  SenseAngle3=off  SenseQ=off  SenseR=off  SenseOmegaX=off  SenseOmegaY=off  SenseOmegaZ=off  SenseOmega1=off  SenseOmega2=off  SenseOmega3=off  SenseQDot=off  SenseRDot=off  SenseAlphaX=off  SenseAlphaY=off  SenseAlphaZ=off  SenseAlpha1=off  SenseAlpha2=off  SenseAlpha3=off  SenseQDDot=off  SenseRDDot=off  SenseX=on  SenseY=on  SenseZ=on  SenseRad=off  SenseAzim=off  SenseDist=off  SenseInc=off  SenseXDot=off  SenseYDot=off  SenseZDot=off  SenseRadDot=off  SenseAzimDot=off  SenseDistDot=off  SenseIncDot=off  SenseXDDot=off  SenseYDDot=off  SenseZDDot=off  SenseRadDDot=off  SenseAzimDDot=off  SenseDistDDot=off  SenseIncDDot=off
  World Frame : sm_lib/Frames and Transforms/World Frame
  Con1_up : PMIOPort  Side=Left
  Con2_down : PMIOPort  Port=2  Side=Left
  Angle_x : Outport
  Angle_y : Outport  Port=2
  wires:
  Sin1/1 -> Angle_y/1
  Sin2/1 -> Angle_x/1
  Sum/1 -> Gain/1
  Gain1/1 -> Product1/1
  Sum3/1 -> Product1/2
  Sum2/1 -> Gain1/1
  Product1/1 -> Sin1/1
  PS-Simulink Converter6/1 -> Sum3/1
  PS-Simulink Converter1/1 -> Sum/2
  PS-Simulink Converter5/1 -> Sum2/2
  PS-Simulink Converter4/1 -> Sum2/1
  PS-Simulink Converter7/1 -> Sum3/2
  Gain/1 -> Product/1
  PS-Simulink Converter3/1 -> Sum1/2
  PS-Simulink Converter2/1 -> Sum1/1
  Product/1 -> Sin2/1
  Sum1/1 -> Product/2
  PS-Simulink Converter/1 -> Sum/1
  connections:
  Con2_down/RConn1 -- Transform Sensor2/RConn1
  Transform Sensor1/RConn1 -- Con1_up/RConn1
  PS-Simulink Converter/LConn1 -- Transform Sensor1/RConn2
  Transform Sensor2/RConn2 -- PS-Simulink Converter1/LConn1
  PS-Simulink Converter4/LConn1 -- Transform Sensor1/RConn3
  PS-Simulink Converter5/LConn1 -- Transform Sensor2/RConn3
  PS-Simulink Converter2/LConn1 -- PS-Simulink Converter6/LConn1 -- Transform Sensor1/RConn4
  PS-Simulink Converter3/LConn1 -- PS-Simulink Converter7/LConn1 -- Transform Sensor2/RConn4
  Transform Sensor1/LConn1 -- Transform Sensor2/LConn1 -- World Frame/RConn1

== system Crane_rigid/All pendulum/Angle sensor 19 ==
  Gain : Gain  Gain=-1
  Gain1 : Gain  Gain=-1
  PS-Simulink Converter{,1..7} (8 alike) : nesl_utility/PS-Simulink Converter  PhysicalDomain=network_engine_domain  SubClassName=ps_output  LeftPortType=input  RightPortType=output  PseudoPeriodic=off  Frequencies=[]  Unit=inherit  AffineConversion=off
      settings: SourceProductBaseCode=PW,SS
  Product : Product  Inputs=*/
  Product1 : Product  Inputs=*/
  Sin1 : Trigonometry  Operator=atan
  Sin2 : Trigonometry  Operator=atan
  Sum{,1..3} (4 alike) : Sum  Inputs=|+-
  Transform Sensor1 : sm_lib/Frames and Transforms/Transform Sensor  MeasurementFrame=World  SenseAngle=off  SenseAxis=off  SenseAngle1=off  SenseAngle2=off  SenseAngle3=off  SenseQ=off  SenseR=off  SenseOmegaX=off  SenseOmegaY=off  SenseOmegaZ=off  SenseOmega1=off  SenseOmega2=off  SenseOmega3=off  SenseQDot=off  SenseRDot=off  SenseAlphaX=off  SenseAlphaY=off  SenseAlphaZ=off  SenseAlpha1=off  SenseAlpha2=off  SenseAlpha3=off  SenseQDDot=off  SenseRDDot=off  SenseX=on  SenseY=on  SenseZ=on  SenseRad=off  SenseAzim=off  SenseDist=off  SenseInc=off  SenseXDot=off  SenseYDot=off  SenseZDot=off  SenseRadDot=off  SenseAzimDot=off  SenseDistDot=off  SenseIncDot=off  SenseXDDot=off  SenseYDDot=off  SenseZDDot=off  SenseRadDDot=off  SenseAzimDDot=off  SenseDistDDot=off  SenseIncDDot=off
  Transform Sensor2 : sm_lib/Frames and Transforms/Transform Sensor  MeasurementFrame=World  SenseAngle=off  SenseAxis=off  SenseAngle1=off  SenseAngle2=off  SenseAngle3=off  SenseQ=off  SenseR=off  SenseOmegaX=off  SenseOmegaY=off  SenseOmegaZ=off  SenseOmega1=off  SenseOmega2=off  SenseOmega3=off  SenseQDot=off  SenseRDot=off  SenseAlphaX=off  SenseAlphaY=off  SenseAlphaZ=off  SenseAlpha1=off  SenseAlpha2=off  SenseAlpha3=off  SenseQDDot=off  SenseRDDot=off  SenseX=on  SenseY=on  SenseZ=on  SenseRad=off  SenseAzim=off  SenseDist=off  SenseInc=off  SenseXDot=off  SenseYDot=off  SenseZDot=off  SenseRadDot=off  SenseAzimDot=off  SenseDistDot=off  SenseIncDot=off  SenseXDDot=off  SenseYDDot=off  SenseZDDot=off  SenseRadDDot=off  SenseAzimDDot=off  SenseDistDDot=off  SenseIncDDot=off
  World Frame : sm_lib/Frames and Transforms/World Frame
  Con1_up : PMIOPort  Side=Left
  Con2_down : PMIOPort  Port=2  Side=Left
  Angle_x : Outport
  Angle_y : Outport  Port=2
  wires:
  PS-Simulink Converter/1 -> Sum/1
  Sum1/1 -> Product/2
  Product/1 -> Sin2/1
  PS-Simulink Converter2/1 -> Sum1/1
  PS-Simulink Converter3/1 -> Sum1/2
  Gain/1 -> Product/1
  PS-Simulink Converter7/1 -> Sum3/2
  PS-Simulink Converter4/1 -> Sum2/1
  PS-Simulink Converter5/1 -> Sum2/2
  PS-Simulink Converter1/1 -> Sum/2
  PS-Simulink Converter6/1 -> Sum3/1
  Product1/1 -> Sin1/1
  Sum2/1 -> Gain1/1
  Sum3/1 -> Product1/2
  Gain1/1 -> Product1/1
  Sum/1 -> Gain/1
  Sin2/1 -> Angle_x/1
  Sin1/1 -> Angle_y/1
  connections:
  World Frame/RConn1 -- Transform Sensor2/LConn1 -- Transform Sensor1/LConn1
  Transform Sensor2/RConn4 -- PS-Simulink Converter7/LConn1 -- PS-Simulink Converter3/LConn1
  Transform Sensor1/RConn4 -- PS-Simulink Converter6/LConn1 -- PS-Simulink Converter2/LConn1
  PS-Simulink Converter5/LConn1 -- Transform Sensor2/RConn3
  PS-Simulink Converter4/LConn1 -- Transform Sensor1/RConn3
  Transform Sensor2/RConn2 -- PS-Simulink Converter1/LConn1
  PS-Simulink Converter/LConn1 -- Transform Sensor1/RConn2
  Transform Sensor1/RConn1 -- Con1_up/RConn1
  Con2_down/RConn1 -- Transform Sensor2/RConn1
